simulink model "E010A5_R2_E1_energy_ton_ramp_40A_1A_20260701_003547"  (R2024b)
settings: Solver=VariableStepAuto  StartTime=0.0  StopTime=0.54e-3  MaxStep=5e-9  RelTol=1e-3
undefined symbols (not defined in the file): A_init, A_lower, A_upper, Cout, DCR_L1, DCR_L2, DCR_L3, DCR_L4, E010_AreaBleed_Enable, E010_AreaHold_Enable, E010_AreaHold_Time, E010_PulseInhibit_Count, E010_PulseInhibit_Enable, E010_PulseInhibit_Time, E010_Reentry_Band_Down, E010_ReentryGuard_Enable, E010_TonTrunc_Enable, E010_Vref, E010A5_DeltaI_Drop_Threshold_High, E010A5_IL_Sense_Gain1, E010A5_IL_Sense_Gain2, E010A5_IL_Sense_Gain3, E010A5_IL_Sense_Gain4, E010A5_R2_BudgetWindow, E010A5_R2_EnergyShaper_Enable, E010A5_R2_FirstTonLimit, E010A5_R2_PreloadTarget, E010A5_R2_ReleaseInitial, E010A5_R2_ReleaseRate, E010A5_R2_ReleaseWindow, E010A5_R2_RestoreRate, E010A5_R2_SchedulerReleaseEnable, E010A5_R2_SecondTonLimit, E010A5_R2_SoftPreloadEnable, E010A5_R2_TonBudget, E010A5_R2_TonRampMax, E010A5_R2_TonRampStep, E010A5_R2_TonRampWindow, E010A5_R2_UndershootBudget, E010A5_R2_UpperReentryBand, E010A5_R2_VoltageWindowEnable, ESR_C, IdealIQCOT_Enable, IL_adc_counts_per_A, IL_pk_limit_adc_neg, IL_pk_limit_adc_pos, Iload_final, Iload_initial, Iph, Iqcot_enable, kappa_cmd, Kiqcot, Kvc_iqcot, L, Lambda0_iqcot, Lambda_m2, rho_cmd, Ri_iqcot, t_load_step, Tblank ... (+18)
libraries: simulink x29, spsCurrentMeasurementLib x8, spsMosfetLib x8, spsSeriesRLCBranchLib x5, spsVoltageMeasurementLib x5, spsDCVoltageSourceLib x4, spsControlledCurrentSourceLib x1, spsGroundLib x1, spspowerguiLib x1
(part 1 of 2)
settings Model: Creator=zengruize  LastModifiedBy=zengruize

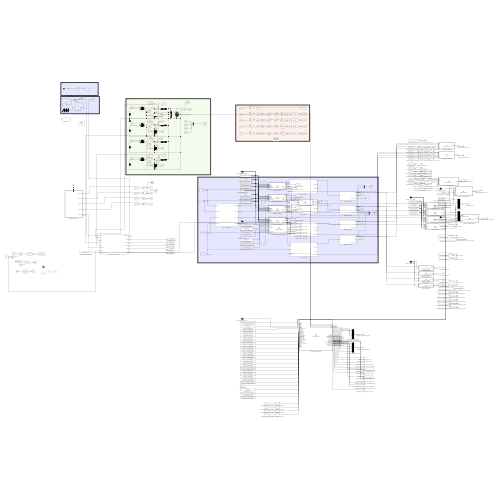
[thumbnail: Simulink's stored preview of the top-level diagram]
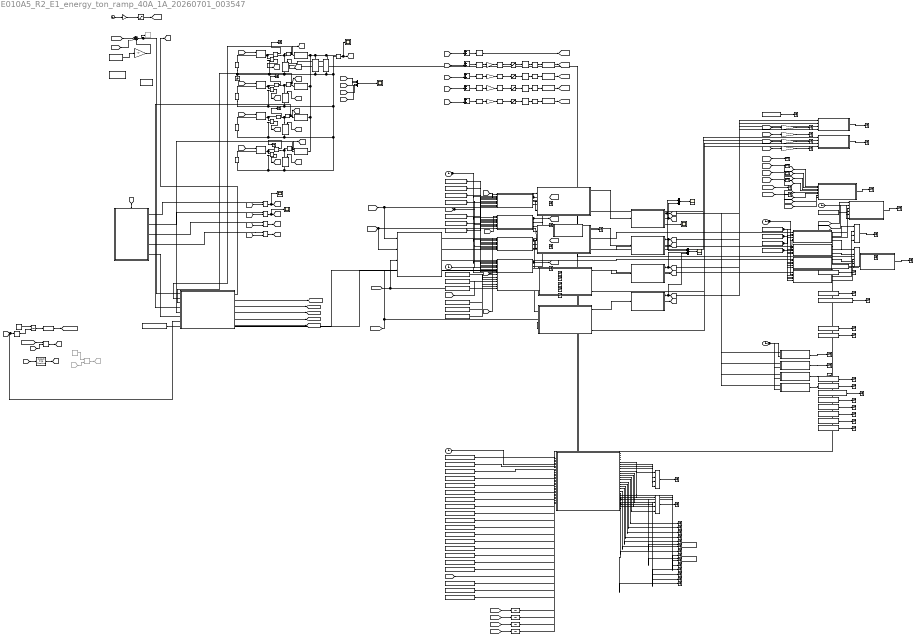
== system E010A5_R2_E1_energy_ton_ramp_40A_1A_20260701_003547 ==
  note: cot
  note: 输出电压误差比较器
  note: 功率级
  note: 软启动
  note: 采样
  Add{,1..4} (5 alike) : Sum
  Bus Creator : BusCreator  Inputs=4
  Bus Creator1 : BusCreator  Inputs=2
  Bus Creator2 : BusCreator  Inputs=4
  COT_Cell_1Phase1 : Subsystem
  COT_Cell_1Phase2 : Subsystem
  COT_Cell_1Phase3 : Subsystem
  COT_Cell_1Phase4 : Subsystem
  Clock : Clock
  Compare To Constant : simulink/Logic and Bit Operations/Compare To Constant  relop=>=  const=Tblank  OutDataTypeStr=boolean
  Constant : Constant
  Current Measurement{,1..3} (4 alike) : spsCurrentMeasurementLib/Current Measurement  PhasorSimulation=off  OutputType=Complex  PSBequivalent=0
  DC Voltage Source{,1..3} (4 alike) : spsDCVoltageSourceLib/DC Voltage Source  Amplitude=Vin  Measurements=None
  Data Type Conversion{,2..4} (4 alike) : DataTypeConversion  OutDataTypeStr=fixdt(1,14,0)  SaturateOnIntegerOverflow=off  RndMeth=Floor
  Detect Rise Positive : simulink/Logic and Bit Operations/Detect Rise Positive  vinit=0  OutDataTypeStr=boolean
  E010A5_ActiveHSPhase : MATLAB Function  TreatAsAtomicUnit=on
  E010A5_ActiveHSPhase_Term : Terminator
  E010A5_AreaBleed_Enable : Constant  Value=E010_AreaBleed_Enable
  E010A5_AreaHold_Bleed_Term : Terminator
  E010A5_AreaHold_Clock : Clock
  E010A5_AreaHold_Count_Term : Terminator
  E010A5_AreaHold_Enable : Constant  Value=E010_AreaHold_Enable
  E010A5_AreaHold_EnableProjection : MATLAB Function  TreatAsAtomicUnit=on  SystemSampleTime=Ts_ctrl
  E010A5_AreaHold_LoadStepTime : Constant  Value=t_load_step
  E010A5_AreaHold_ReentryBand : Constant  Value=E010_Reentry_Band_Down
  E010A5_AreaHold_Reset_Term : Terminator
  E010A5_AreaHold_State_Term : Terminator
  E010A5_AreaHold_Time : Constant  Value=E010_AreaHold_Time
  E010A5_AreaHold_Vref : Constant  Value=E010_Vref
  E010A5_CurrentLimitHit : MATLAB Function  TreatAsAtomicUnit=on
  E010A5_CurrentLimitHit_Term : Terminator
  E010A5_IL_Sense_Gain_Block1 : Gain  Gain=E010A5_IL_Sense_Gain1
  E010A5_IL_Sense_Gain_Block2 : Gain  Gain=E010A5_IL_Sense_Gain2
  E010A5_IL_Sense_Gain_Block3 : Gain  Gain=E010A5_IL_Sense_Gain3
  E010A5_IL_Sense_Gain_Block4 : Gain  Gain=E010A5_IL_Sense_Gain4
  E010A5_IL_Sense_Term{1..4} (4 alike) : Terminator
  E010A5_LoadCurrentStep : Step  Time=t_load_step  Before=Iload_initial  After=Iload_final  SampleTime=0
  E010A5_Load_Current_Source : spsControlledCurrentSourceLib/Controlled Current Source  Initialize=on  Source_Type=DC  Amplitude=0  Phase=0  Frequency=0  Measurements=None
  E010A5_Log_Lambda_i_Term : Terminator
  E010A5_Log_REQ1_Term : Terminator
  E010A5_Log_REQ2_Term : Terminator
  E010A5_Log_REQ3_Term : Terminator
  E010A5_Log_REQ4_Term : Terminator
  E010A5_Log_area_int_i_Term : Terminator
  E010A5_PhaseOrderError : MATLAB Function  TreatAsAtomicUnit=on  SystemSampleTime=Ts_ctrl
  E010A5_PhaseOrderError_Term : Terminator
  E010A5_PhaseOrder_Clock : Clock
  E010A5_PhaseOrder_LoadStepTime : Constant  Value=t_load_step
  E010A5_PulseInhibit1 : MATLAB Function  TreatAsAtomicUnit=on
  E010A5_PulseInhibit1_Count_Term : Terminator
  E010A5_PulseInhibit2 : MATLAB Function  TreatAsAtomicUnit=on
  E010A5_PulseInhibit2_Count_Term : Terminator
  E010A5_PulseInhibit3 : MATLAB Function  TreatAsAtomicUnit=on
  E010A5_PulseInhibit3_Count_Term : Terminator
  E010A5_PulseInhibit4 : MATLAB Function  TreatAsAtomicUnit=on
  E010A5_PulseInhibit4_Count_Term : Terminator
  E010A5_PulseInhibitState : MATLAB Function  TreatAsAtomicUnit=on
  E010A5_PulseInhibitState_Term : Terminator
  E010A5_PulseInhibit_Clock : Clock
  E010A5_PulseInhibit_Count : Constant  Value=E010_PulseInhibit_Count
  E010A5_PulseInhibit_Enable : Constant  Value=E010_PulseInhibit_Enable
  E010A5_PulseInhibit_LoadStepTime : Constant  Value=t_load_step
  E010A5_PulseInhibit_ReentryBand : Constant  Value=E010_Reentry_Band_Down
  E010A5_PulseInhibit_ReentryGuard : Constant  Value=E010_ReentryGuard_Enable
  E010A5_PulseInhibit_Time : Constant  Value=E010_PulseInhibit_Time
  E010A5_PulseInhibit_Vref : Constant  Value=E010_Vref
  E010A5_R2_BudgetWindow : Constant  Value=E010A5_R2_BudgetWindow
  E010A5_R2_EnergyShaper : MATLAB Function  TreatAsAtomicUnit=on  SystemSampleTime=Tss
  E010A5_R2_Energy_Clock : Clock
  E010A5_R2_Energy_Enable : Constant  Value=E010A5_R2_EnergyShaper_Enable
  E010A5_R2_FirstTonLimit : Constant  Value=E010A5_R2_FirstTonLimit
  E010A5_R2_LoadStepTime : Constant  Value=t_load_step
  E010A5_R2_PreloadTarget : Constant  Value=E010A5_R2_PreloadTarget
  E010A5_R2_REQAccept_Delay{1..4} (4 alike) : UnitDelay  SampleTime=Tss  HasFrameUpgradeWarning=on
  E010A5_R2_ReleaseInitial : Constant  Value=E010A5_R2_ReleaseInitial
  E010A5_R2_ReleaseRate : Constant  Value=E010A5_R2_ReleaseRate
  E010A5_R2_ReleaseWindow : Constant  Value=E010A5_R2_ReleaseWindow
  E010A5_R2_RestoreRate : Constant  Value=E010A5_R2_RestoreRate
  E010A5_R2_SchedulerReleaseEnable : Constant  Value=E010A5_R2_SchedulerReleaseEnable
  E010A5_R2_SecondTonLimit : Constant  Value=E010A5_R2_SecondTonLimit
  E010A5_R2_SoftPreloadEnable : Constant  Value=E010A5_R2_SoftPreloadEnable
  E010A5_R2_TonBudget : Constant  Value=E010A5_R2_TonBudget
  E010A5_R2_TonRampLimit_Mux : Mux
  E010A5_R2_TonRampLimit_Term : Terminator
  E010A5_R2_TonRampMax : Constant  Value=E010A5_R2_TonRampMax
  E010A5_R2_TonRampStep : Constant  Value=E010A5_R2_TonRampStep
  E010A5_R2_TonRampUsage_Mux : Mux
  E010A5_R2_TonRampUsage_Term : Terminator
  E010A5_R2_TonRampWindow : Constant  Value=E010A5_R2_TonRampWindow
  E010A5_R2_Ton_ramp_state_Term : Terminator
  E010A5_R2_UndershootBudget : Constant  Value=E010A5_R2_UndershootBudget
  E010A5_R2_UpperBand : Constant  Value=E010A5_R2_UpperReentryBand
  E010A5_R2_VoltageWindowEnable : Constant  Value=E010A5_R2_VoltageWindowEnable
  E010A5_R2_Vref : Constant  Value=E010_Vref
  E010A5_R2_area_int_restore_state_Term : Terminator
  E010A5_R2_area_int_soft_preload_count_Term : Terminator
  E010A5_R2_area_int_soft_preload_state_Term : Terminator
  E010A5_R2_controlled_reentry_active_Term : Terminator
  E010A5_R2_energy_budget_state_Term : Terminator
  E010A5_R2_reentry_energy_budget_remaining_Term : Terminator
  E010A5_R2_reentry_energy_budget_used_Term : Terminator
  E010A5_R2_reentry_energy_budget_violation_Term : Terminator
  E010A5_R2_scheduler_release_fraction_Term : Terminator
  E010A5_R2_scheduler_release_guard_violation_Term : Terminator
  E010A5_R2_scheduler_release_state_Term : Terminator
  E010A5_R2_voltage_window_release_state_Term : Terminator
  E010A5_R2_voltage_window_release_violation_Term : Terminator
  E010A5_REQRejectReason : MATLAB Function  TreatAsAtomicUnit=on
  E010A5_REQRejectReason_Term : Terminator
  E010A5_Reentry_State_Term : Terminator
  E010A5_SevereDropDetector : MATLAB Function  TreatAsAtomicUnit=on  SystemSampleTime=Ts_ctrl
  E010A5_SevereDropDetector_Clock : Clock
  E010A5_SevereDropDetector_Term : Terminator
  E010A5_SevereDropThreshold : Constant  Value=E010A5_DeltaI_Drop_Threshold_High
  E010A5_TonActual1 : MATLAB Function  TreatAsAtomicUnit=on  SystemSampleTime=Ts_ctrl
  E010A5_TonActual1_Term : Terminator
  E010A5_TonActual2 : MATLAB Function  TreatAsAtomicUnit=on  SystemSampleTime=Ts_ctrl
  E010A5_TonActual2_Term : Terminator
  E010A5_TonActual3 : MATLAB Function  TreatAsAtomicUnit=on  SystemSampleTime=Ts_ctrl
  E010A5_TonActual3_Term : Terminator
  E010A5_TonActual4 : MATLAB Function  TreatAsAtomicUnit=on  SystemSampleTime=Ts_ctrl
  E010A5_TonActual4_Term : Terminator
  E010A5_TonActual_Clock : Clock
  E010A5_TonSaved_Mux : Mux
  E010A5_TonSaved_Term : Terminator
  E010A5_TonTrunc1 : MATLAB Function  TreatAsAtomicUnit=on
  E010A5_TonTrunc2 : MATLAB Function  TreatAsAtomicUnit=on
  E010A5_TonTrunc3 : MATLAB Function  TreatAsAtomicUnit=on
  E010A5_TonTrunc4 : MATLAB Function  TreatAsAtomicUnit=on
  E010A5_TonTrunc_Clock : Clock
  E010A5_TonTrunc_Enable : Constant  Value=E010_TonTrunc_Enable
  E010A5_TonTrunc_LoadStepTime : Constant  Value=t_load_step
  E010A5_TonTrunc_Min : Constant  Value=Tton_trunc_min
  E010A5_TonTrunc_Mux : Mux
  E010A5_TonTrunc_Term : Terminator
  E010A5_TonTrunc_Window : Constant  Value=Tton_trunc_window
  E010A5_Ton_nom : Constant  Value=Ton_nom
  E010A5_Ton_nom_Term : Terminator
  E010A5_a_O_state : Constant  Value=71
  E010A5_a_O_state_Term : Terminator
  E010A5_active_phase_set : Constant  Value=[1 1 1 1]
  E010A5_active_phase_set_Term : Terminator
  E010A5_area_int_reentry_clamp : Constant  Value=0
  E010A5_area_int_reentry_clamp_Term : Terminator
  E010A5_burst_limiter_clamp_count : Constant  Value=0
  E010A5_burst_limiter_clamp_count_Term : Terminator
  E010A5_burst_limiter_fallback_reason : Constant  Value=0
  E010A5_burst_limiter_fallback_reason_Term : Terminator
  E010A5_burst_limiter_release_count : Constant  Value=0
  E010A5_burst_limiter_release_count_Term : Terminator
  E010A5_burst_limiter_state : Constant  Value=0
  E010A5_burst_limiter_state_Term : Terminator
  E010A5_burst_pulse_count_after_reentry : Constant  Value=0
  E010A5_burst_pulse_count_after_reentry_Term : Terminator
  E010A5_fallback_count : Constant  Value=0
  E010A5_fallback_count_Term : Terminator
  E010A5_fallback_reason : Constant  Value=0
  E010A5_fallback_reason_Term : Terminator
  E010A5_fallback_state : Constant  Value=0
  E010A5_fallback_state_Term : Terminator
  E010A5_recovery_Ton_ramp_usage : Constant  Value=0
  E010A5_recovery_Ton_ramp_usage_Term : Terminator
  E010A5_scheduler_release_gate_active : Constant  Value=0
  E010A5_scheduler_release_gate_active_Term : Terminator
  From31 : From  Commented=on  GotoTag=REQ
  Gain : Gain  Gain=Vo_ref / Tss
  Gain11 : Gain  Gain=205
  Gain12 : Gain  Gain=-205
  Gain13 : Gain  Gain=205
  Gain9 : Gain  Gain=-205
  GateDriver_1Phase1 : Subsystem
  GateDriver_1Phase2 : Subsystem
  GateDriver_1Phase3 : Subsystem
  GateDriver_1Phase4 : Subsystem
  Goto26 : Goto  Commented=on  GotoTag=tr
  Ground : spsGroundLib/Ground  LConnTagsString=a
  IHS_Terminator{1..4} (4 alike) : Terminator
  IL_Measurement{1..4} (4 alike) : spsCurrentMeasurementLib/Current Measurement  PhasorSimulation=off  OutputType=Complex  PSBequivalent=0
  IQCOT_Ton_Adapter : Subsystem
  IdealIQCOT_Enable_Constant : Constant  Value=IdealIQCOT_Enable
  Ideal_Digital_IQCOT_Request : Subsystem
  Integrator : Integrator  ExternalReset=rising
  Logical Operator{,1..4} (5 alike) : Logic  AllPortsSameDT=off  OutDataTypeStr=boolean
  Logical Operator5 : Logic  Commented=on  AllPortsSameDT=off  OutDataTypeStr=boolean
  Memory : Memory
  Mosfet{,1..3} (4 alike) : spsMosfetLib/Mosfet  Ron=Ron_HS  Lon=0  Rd=Rd_body  Vfd=Vfd_body  IC=0  Rs=Rs_snubber  Cs=Cs_snubber  Measurements=on
  Mosfet{4..7} (4 alike) : spsMosfetLib/Mosfet  Ron=Ron_LS  Lon=0  Rd=Rd_body  Vfd=Vfd_body  IC=0  Rs=Rs_snubber  Cs=Cs_snubber  Measurements=on
  OnDelay : Subsystem
  PhaseScheduler_4Phase : Subsystem  TreatAsAtomicUnit=on
  Pulse Generator : DiscretePulseGenerator  Commented=on  PulseType=Time based  Period=Tblank  PulseWidth=5
  Quantizer{1..4} (4 alike) : Quantizer  QuantizationInterval=1
  Relay : Relay  Commented=through  OnSwitchValue=Vhys/2  OffSwitchValue=-Vhys/2
  Saturation{,1,3..4} (4 alike) : Saturate  UpperLimit=8191  LowerLimit=-8191
  Saturation2 : Saturate  UpperLimit=Vo_ref  LowerLimit=0
  Scope{,1..6} (7 alike) : Scope
  Series RLC Branch : spsSeriesRLCBranchLib/Series RLC Branch  LConnTagsString=__new0  RConnTagsString=__new0  BranchType=RL  Resistance=DCR_L1  Inductance=L  SetiL0=off  InitialCurrent=0  Capacitance=1e-6  Setx0=off  InitialVoltage=0  Measurements=None
  Series RLC Branch1 : spsSeriesRLCBranchLib/Series RLC Branch  LConnTagsString=__new0  RConnTagsString=__new0  BranchType=RL  Resistance=DCR_L2  Inductance=L  SetiL0=off  InitialCurrent=0  Capacitance=1e-6  Setx0=off  InitialVoltage=0  Measurements=None
  Series RLC Branch2 : spsSeriesRLCBranchLib/Series RLC Branch  LConnTagsString=__new0  RConnTagsString=__new0  BranchType=RL  Resistance=DCR_L3  Inductance=L  SetiL0=off  InitialCurrent=0  Capacitance=1e-6  Setx0=off  InitialVoltage=0  Measurements=None
  Series RLC Branch3 : spsSeriesRLCBranchLib/Series RLC Branch  LConnTagsString=__new0  RConnTagsString=__new0  BranchType=RL  Resistance=DCR_L4  Inductance=L  SetiL0=off  InitialCurrent=0  Capacitance=1e-6  Setx0=off  InitialVoltage=0  Measurements=None
  Series RLC Branch4 : spsSeriesRLCBranchLib/Series RLC Branch  LConnTagsString=__new0  RConnTagsString=__new0  BranchType=RC  Resistance=ESR_C  Inductance=1e-3  SetiL0=off  InitialCurrent=0  Capacitance=Cout  Setx0=on  InitialVoltage=Vo_ref  Measurements=None
  Sum : Sum  Inputs=|+--
  Transport Delay{1..4} (4 alike) : TransportDelay  DelayTime=5/25000000
  VCOT_Ramp_Gain : Gain  Gain=Vcot_ramp_enable * Vcot_ramp_amp
  VCOT_Ramp_Unit : simulink/Sources/Repeating Sequence  rep_seq_t=[0 Tslot]  rep_seq_y=[0 1]
  Voltage Measurement{,1..4} (5 alike) : spsVoltageMeasurementLib/Voltage Measurement  PhasorSimulation=off  OutputType=Complex  PSBequivalent=0
  Zero-Order Hold{1..4,19..23} (9 alike) : ZeroOrderHold  SampleTime=1/25000000
  powergui : spspowerguiLib/powergui  Priority=1  SimulationMode=Discrete  SampleTime=2e-9  frequency=60  Iterations=50  frequencyindice=0  Pbase=100e6  ErrMax=1e-4  UnitsV=kV  UnitsW=MW  buscounter=0  FunctionMessages=off  echomessages=off  EnableUseOfTLC=off  CurrentSourceSwitches=off  DisableSnubberDevices=off  DisableRonSwitches=off  DisableVfSwitches=off  DisplayEquations=off  AutomaticDiscreteSolvers=off  SolverType=Tustin/Backward Euler (TBE)  Interpol=off  ExternalGateDelay=off  methode=off  Ts=100  x0status=blocks  SPID=on  SwTol=0  HookPort=off  NonlinearTolerance=1e-4  nMaxIteration=100  ContinueOnMaxIteration=off  RestoreLinks=warning  ResistiveCurrentMeasurement=off  Frange=[0:2:500]  Ylog=off  Xlog=on  ShowGrid=off  save=off  variable=ZData  structure=0  ZoomFFT=off  StartTime=0.0  cycles=1  DisplayStyle=1  fundamental=60  FreqAxis=off  MaxFrequency=1000  frequencyindicesteady=1  RmsSteady=1  display=off
  wires:
  [QH1] -> Mosfet/1
  [QH4] -> Mosfet3/1
  [QH2] -> Mosfet1/1
  [QH3] -> Mosfet2/1
  [QL1] -> Mosfet4/1
  [QL2] -> Mosfet5/1
  [QL3] -> Mosfet6/1
  [QL4] -> Mosfet7/1
  Voltage Measurement2/1 -> [SW2]  "SW2"
  Voltage Measurement3/1 -> [SW3]  "SW3"
  Voltage Measurement1/1 -> [SW1]  "SW1"
  Voltage Measurement4/1 -> [SW4]  "SW4"
  GateDriver_1Phase1/1(QHi) -> Bus Creator1/1, [QH1], Bus Creator2/1, E010A5_ActiveHSPhase/1(qh1), E010A5_TonActual1/1(qh)  "QH1"
  GateDriver_1Phase2/1(QHi) -> Bus Creator2/2, [QH2], E010A5_ActiveHSPhase/2(qh2), E010A5_TonActual2/1(qh)  "QH2"
  GateDriver_1Phase3/1(QHi) -> Bus Creator2/3, [QH3], E010A5_ActiveHSPhase/3(qh3), E010A5_TonActual3/1(qh)  "QH3"
  GateDriver_1Phase4/1(QHi) -> Bus Creator2/4, [QH4], E010A5_ActiveHSPhase/4(qh4), E010A5_TonActual4/1(qh)  "QH4"
  GateDriver_1Phase1/2(QLi) -> Bus Creator1/2, [QL1]  "QL1"
  GateDriver_1Phase2/2(QLi) -> [QL2]  "QL2"
  GateDriver_1Phase3/2(QLi) -> [QL3]  "QL3"
  GateDriver_1Phase4/2(QLi) -> [QL4]  "QL4"
  COT_Cell_1Phase1/1(Qi) -> GateDriver_1Phase1/1(Qi)
  COT_Cell_1Phase2/1(Qi) -> GateDriver_1Phase2/1(Qi)
  COT_Cell_1Phase3/1(Qi) -> GateDriver_1Phase3/1(Qi)
  COT_Cell_1Phase4/1(Qi) -> GateDriver_1Phase4/1(Qi)
  GateDriver_1Phase1/3(ShootThrough_i) -> Scope1/1
  Bus Creator/1 -> Scope2/1
  [SW1] -> Bus Creator/1
  [SW2] -> Bus Creator/2
  [SW3] -> Bus Creator/3
  [SW4] -> Bus Creator/4
  Bus Creator1/1 -> Scope3/1
  Saturation2/1 -> [Vref_soft]
  Gain/1 -> Saturation2/1
  Clock/1 -> Gain/1
  Voltage Measurement/1 -> Scope/1, [Vout]  "Vout"
  [Vref_soft] -> Sum/1
  [Vo_sample] -> Sum/2
  Sum/1 -> Ideal_Digital_IQCOT_Request/1(e_v), Relay/1  "e_v"
  Constant/1 -> Integrator/1
  Integrator/1 -> Compare To Constant/1
  Compare To Constant/1 -> [GlobalReady]  "Allow"
  [GlobalReady] -> Logical Operator/1
  [REQ] -> Logical Operator/2
  Logical Operator/1 -> [Allow]
  [Allow] -> Detect Rise Positive/1
  Detect Rise Positive/1 -> [tr]
  [tr] -> PhaseScheduler_4Phase/Trigger  "tr"
  PhaseScheduler_4Phase/1(phase_en1) -> Logical Operator1/1
  [tr] -> Logical Operator1/2
  PhaseScheduler_4Phase/2(phase_en2) -> Logical Operator2/1
  [tr] -> Logical Operator2/2
  PhaseScheduler_4Phase/3(phase_en3) -> Logical Operator3/1
  [tr] -> Logical Operator3/2
  PhaseScheduler_4Phase/4(phase_en4) -> Logical Operator4/1
  [tr] -> Logical Operator4/2
  Logical Operator1/1 -> Scope4/1, [tr1]  "tr1"
  Logical Operator2/1 -> Scope5/1, [tr2]  "tr2"
  Logical Operator3/1 -> [tr3]  "tr3"
  Logical Operator4/1 -> [tr4]  "tr4"
  [IL_sample1] -> COT_Cell_1Phase1/2(ILi), IQCOT_Ton_Adapter/1(IL_sample1)  "IL_sample1"
  [IL_sample2] -> IQCOT_Ton_Adapter/2(IL_sample2), COT_Cell_1Phase2/2(ILi)  "IL_sample2"
  [IL_sample3] -> IQCOT_Ton_Adapter/3(IL_sample3), COT_Cell_1Phase3/2(ILi)  "IL_sample3"
  [IL_sample4] -> IQCOT_Ton_Adapter/4(IL_sample4), COT_Cell_1Phase4/2(ILi)  "IL_sample4"
  [tr] -> Memory/1, Ideal_Digital_IQCOT_Request/7(tr_reset)  "tr_reset"
  Memory/1 -> Integrator/2
  Logical Operator5/1 -> Goto26/1
  Pulse Generator/1 -> Logical Operator5/1
  From31/1 -> Logical Operator5/2
  Bus Creator2/1 -> Scope6/1
  IL_Measurement1/1 -> [IL1], Ideal_Digital_IQCOT_Request/2(IL1)  "IL1"
  IL_Measurement2/1 -> [IL2], Ideal_Digital_IQCOT_Request/3(IL2)  "IL2"
  IL_Measurement3/1 -> [IL3], Ideal_Digital_IQCOT_Request/4(IL3)  "IL3"
  IL_Measurement4/1 -> [IL4], Ideal_Digital_IQCOT_Request/5(IL4)  "IL4"
  Current Measurement/1 -> IHS_Terminator1/1
  Current Measurement1/1 -> IHS_Terminator2/1
  Current Measurement2/1 -> IHS_Terminator3/1
  Current Measurement3/1 -> IHS_Terminator4/1
  Zero-Order Hold23/1 -> Gain13/1
  Zero-Order Hold20/1 -> Gain9/1
  Zero-Order Hold3/1 -> Data Type Conversion3/1
  Zero-Order Hold4/1 -> Data Type Conversion2/1
  Saturation4/1 -> Transport Delay4/1
  Zero-Order Hold1/1 -> Data Type Conversion/1
  [IL3] -> Add3/2
  Add3/1 -> Zero-Order Hold22/1
  Quantizer1/1 -> Saturation/1
  Quantizer4/1 -> Saturation4/1
  Gain12/1 -> Quantizer3/1
  [IL4] -> Add4/2
  Add/1 -> Zero-Order Hold19/1
  Data Type Conversion/1 -> [IL_sample1]
  Data Type Conversion2/1 -> [IL_sample4]
  Add4/1 -> Zero-Order Hold23/1
  Transport Delay3/1 -> Zero-Order Hold3/1
  Saturation3/1 -> Transport Delay3/1
  Add1/1 -> Zero-Order Hold20/1
  [IL1] -> Add1/2
  Transport Delay4/1 -> Zero-Order Hold4/1
  Zero-Order Hold21/1 -> Gain11/1
  Data Type Conversion3/1 -> [IL_sample3]
  Gain9/1 -> Quantizer1/1
  Gain11/1 -> Quantizer2/1
  Saturation/1 -> Transport Delay1/1
  [IL2] -> Add2/2
  Transport Delay2/1 -> Zero-Order Hold2/1
  Zero-Order Hold19/1 -> [Vo_sample]
  Gain13/1 -> Quantizer4/1
  Quantizer3/1 -> Saturation3/1
  Data Type Conversion4/1 -> [IL_sample2]
  Zero-Order Hold2/1 -> Data Type Conversion4/1
  Add2/1 -> Zero-Order Hold21/1
  Transport Delay1/1 -> Zero-Order Hold1/1
  [Vout] -> Add/2
  Saturation1/1 -> Transport Delay2/1
  Zero-Order Hold22/1 -> Gain12/1
  Quantizer2/1 -> Saturation1/1
  VCOT_Ramp_Unit/1 -> VCOT_Ramp_Gain/1
  VCOT_Ramp_Gain/1 -> Sum/3  "Vcot_ramp"
  PhaseScheduler_4Phase/5(phase_idx) -> Ideal_Digital_IQCOT_Request/6(phase_idx)  "phase_idx"
  Ideal_Digital_IQCOT_Request/1(REQ_iqcot) -> [REQ]  "REQ_iqcot"
  Ideal_Digital_IQCOT_Request/2(A_iqcot) -> [A_iqcot]  "A_iqcot"
  Ideal_Digital_IQCOT_Request/3(Lambda_i) -> [Lambda_i]  "Lambda_i"
  Ideal_Digital_IQCOT_Request/4(h_iqcot) -> [h_iqcot]  "h_iqcot"
  Ideal_Digital_IQCOT_Request/5(IL_sel) -> [IL_sel]  "IL_sel"
  Ideal_Digital_IQCOT_Request/6(vc_ctrl) -> [vc_ctrl]  "vc_ctrl"
  E010A5_LoadCurrentStep/1 -> E010A5_Load_Current_Source/1, E010A5_SevereDropDetector/1(iload)  "Iload"
  E010A5_active_phase_set/1 -> E010A5_active_phase_set_Term/1  "active_phase_set"
  [IL1] -> E010A5_IL_Sense_Gain_Block1/1
  E010A5_IL_Sense_Gain_Block1/1 -> E010A5_IL_Sense_Term1/1  "IL_sense1"
  [IL2] -> E010A5_IL_Sense_Gain_Block2/1
  E010A5_IL_Sense_Gain_Block2/1 -> E010A5_IL_Sense_Term2/1  "IL_sense2"
  [IL3] -> E010A5_IL_Sense_Gain_Block3/1
  E010A5_IL_Sense_Gain_Block3/1 -> E010A5_IL_Sense_Term3/1  "IL_sense3"
  [IL4] -> E010A5_IL_Sense_Gain_Block4/1
  E010A5_IL_Sense_Gain_Block4/1 -> E010A5_IL_Sense_Term4/1  "IL_sense4"
  [tr1] -> E010A5_Log_REQ1_Term/1  "REQ1"
  [tr2] -> E010A5_Log_REQ2_Term/1  "REQ2"
  [tr3] -> E010A5_Log_REQ3_Term/1  "REQ3"
  [tr4] -> E010A5_Log_REQ4_Term/1  "REQ4"
  [Lambda_i] -> E010A5_Log_Lambda_i_Term/1  "Lambda_i"
  [A_iqcot] -> E010A5_Log_area_int_i_Term/1  "area_int_i"
  E010A5_ActiveHSPhase/1(active_phase) -> E010A5_ActiveHSPhase_Term/1  "active_HS_phase"
  COT_Cell_1Phase1/4(CurrentLimit_i) -> E010A5_CurrentLimitHit/1(u1)
  COT_Cell_1Phase2/4(CurrentLimit_i) -> E010A5_CurrentLimitHit/2(u2)
  COT_Cell_1Phase3/4(CurrentLimit_i) -> E010A5_CurrentLimitHit/3(u3)
  COT_Cell_1Phase4/4(CurrentLimit_i) -> E010A5_CurrentLimitHit/4(u4)
  E010A5_CurrentLimitHit/1(y) -> E010A5_CurrentLimitHit_Term/1  "current_limit_hit"
  IQCOT_Ton_Adapter/1(Ton_iqcot1) -> E010A5_TonTrunc1/1(ton_in)  "Ton_iqcot1"
  E010A5_TonTrunc_Clock/1 -> E010A5_TonTrunc1/2(t), E010A5_TonTrunc2/2(t), E010A5_TonTrunc3/2(t), E010A5_TonTrunc4/2(t)
  E010A5_TonTrunc_LoadStepTime/1 -> E010A5_TonTrunc1/3(t_step), E010A5_TonTrunc2/3(t_step), E010A5_TonTrunc3/3(t_step), E010A5_TonTrunc4/3(t_step)
  E010A5_TonTrunc_Window/1 -> E010A5_TonTrunc1/4(t_window), E010A5_TonTrunc2/4(t_window), E010A5_TonTrunc3/4(t_window), E010A5_TonTrunc4/4(t_window)
  E010A5_TonTrunc_Min/1 -> E010A5_TonTrunc1/5(t_min), E010A5_TonTrunc2/5(t_min), E010A5_TonTrunc3/5(t_min), E010A5_TonTrunc4/5(t_min)
  E010A5_TonTrunc_Enable/1 -> E010A5_TonTrunc1/6(enable), E010A5_TonTrunc2/6(enable), E010A5_TonTrunc3/6(enable), E010A5_TonTrunc4/6(enable)
  E010A5_TonTrunc1/1(ton_out) -> E010A5_R2_EnergyShaper/1(ton1)  "Ton_cmd1"
  E010A5_TonTrunc1/2(trunc_active) -> E010A5_TonTrunc_Mux/1
  E010A5_TonTrunc1/3(ton_saved) -> E010A5_TonSaved_Mux/1
  IQCOT_Ton_Adapter/2(Ton_iqcot2) -> E010A5_TonTrunc2/1(ton_in)  "Ton_iqcot2"
  E010A5_TonTrunc2/1(ton_out) -> E010A5_R2_EnergyShaper/2(ton2)  "Ton_cmd2"
  E010A5_TonTrunc2/2(trunc_active) -> E010A5_TonTrunc_Mux/2
  E010A5_TonTrunc2/3(ton_saved) -> E010A5_TonSaved_Mux/2
  IQCOT_Ton_Adapter/3(Ton_iqcot3) -> E010A5_TonTrunc3/1(ton_in)  "Ton_iqcot3"
  E010A5_TonTrunc3/1(ton_out) -> E010A5_R2_EnergyShaper/3(ton3)  "Ton_cmd3"
  E010A5_TonTrunc3/2(trunc_active) -> E010A5_TonTrunc_Mux/3
  E010A5_TonTrunc3/3(ton_saved) -> E010A5_TonSaved_Mux/3
  IQCOT_Ton_Adapter/4(Ton_iqcot4) -> E010A5_TonTrunc4/1(ton_in)  "Ton_iqcot4"
  E010A5_TonTrunc4/1(ton_out) -> E010A5_R2_EnergyShaper/4(ton4)  "Ton_cmd4"
  E010A5_TonTrunc4/2(trunc_active) -> E010A5_TonTrunc_Mux/4
  E010A5_TonTrunc4/3(ton_saved) -> E010A5_TonSaved_Mux/4
  E010A5_TonTrunc_Mux/1 -> E010A5_TonTrunc_Term/1  "Ton_trunc_i"
  E010A5_TonSaved_Mux/1 -> E010A5_TonSaved_Term/1  "Ton_saved_i"
  [tr1] -> E010A5_PulseInhibit1/1(tr_in)
  E010A5_PulseInhibit_Clock/1 -> E010A5_PulseInhibit1/2(t), E010A5_PulseInhibit2/2(t), E010A5_PulseInhibit3/2(t), E010A5_PulseInhibit4/2(t)
  E010A5_PulseInhibit_LoadStepTime/1 -> E010A5_PulseInhibit1/3(t_step), E010A5_PulseInhibit2/3(t_step), E010A5_PulseInhibit3/3(t_step), E010A5_PulseInhibit4/3(t_step)
  E010A5_PulseInhibit_Time/1 -> E010A5_PulseInhibit1/4(t_window), E010A5_PulseInhibit2/4(t_window), E010A5_PulseInhibit3/4(t_window), E010A5_PulseInhibit4/4(t_window)
  E010A5_PulseInhibit_Count/1 -> E010A5_PulseInhibit1/5(count_max), E010A5_PulseInhibit2/5(count_max), E010A5_PulseInhibit3/5(count_max), E010A5_PulseInhibit4/5(count_max)
  E010A5_PulseInhibit_Enable/1 -> E010A5_PulseInhibit1/6(enable), E010A5_PulseInhibit2/6(enable), E010A5_PulseInhibit3/6(enable), E010A5_PulseInhibit4/6(enable)
  [Vout] -> E010A5_PulseInhibit1/7(vout), E010A5_PulseInhibit2/7(vout), E010A5_PulseInhibit3/7(vout), E010A5_PulseInhibit4/7(vout)
  E010A5_PulseInhibit_Vref/1 -> E010A5_PulseInhibit1/8(vref), E010A5_PulseInhibit2/8(vref), E010A5_PulseInhibit3/8(vref), E010A5_PulseInhibit4/8(vref)
  E010A5_PulseInhibit_ReentryBand/1 -> E010A5_PulseInhibit1/9(reentry_band), E010A5_PulseInhibit2/9(reentry_band), E010A5_PulseInhibit3/9(reentry_band), E010A5_PulseInhibit4/9(reentry_band)
  E010A5_PulseInhibit_ReentryGuard/1 -> E010A5_PulseInhibit1/10(guard_enable), E010A5_PulseInhibit2/10(guard_enable), E010A5_PulseInhibit3/10(guard_enable), E010A5_PulseInhibit4/10(guard_enable)
  E010A5_PulseInhibit1/1(tr_out) -> COT_Cell_1Phase1/1(tri), [REQ_accept1]  "REQ_accept1"
  E010A5_PulseInhibit1/2(inhibit_active) -> E010A5_PulseInhibitState/1(u1)
  E010A5_PulseInhibit1/3(inhibit_count) -> E010A5_PulseInhibit1_Count_Term/1  "pulse_inhibit_count1"
  [tr2] -> E010A5_PulseInhibit2/1(tr_in)
  E010A5_PulseInhibit2/1(tr_out) -> COT_Cell_1Phase2/1(tri), [REQ_accept2]  "REQ_accept2"
  E010A5_PulseInhibit2/2(inhibit_active) -> E010A5_PulseInhibitState/2(u2)
  E010A5_PulseInhibit2/3(inhibit_count) -> E010A5_PulseInhibit2_Count_Term/1  "pulse_inhibit_count2"
  [tr3] -> E010A5_PulseInhibit3/1(tr_in)
  E010A5_PulseInhibit3/1(tr_out) -> COT_Cell_1Phase3/1(tri), [REQ_accept3]  "REQ_accept3"
  E010A5_PulseInhibit3/2(inhibit_active) -> E010A5_PulseInhibitState/3(u3)
  E010A5_PulseInhibit3/3(inhibit_count) -> E010A5_PulseInhibit3_Count_Term/1  "pulse_inhibit_count3"
  [tr4] -> E010A5_PulseInhibit4/1(tr_in)
  E010A5_PulseInhibit4/1(tr_out) -> COT_Cell_1Phase4/1(tri), [REQ_accept4]  "REQ_accept4"
  E010A5_PulseInhibit4/2(inhibit_active) -> E010A5_PulseInhibitState/4(u4)
  E010A5_PulseInhibit4/3(inhibit_count) -> E010A5_PulseInhibit4_Count_Term/1  "pulse_inhibit_count4"
  E010A5_PulseInhibitState/1(y) -> E010A5_PulseInhibitState_Term/1  "pulse_inhibit_state"
  IdealIQCOT_Enable_Constant/1 -> E010A5_AreaHold_EnableProjection/1(enable_in)
  E010A5_AreaHold_Clock/1 -> E010A5_AreaHold_EnableProjection/2(t)
  E010A5_AreaHold_LoadStepTime/1 -> E010A5_AreaHold_EnableProjection/3(t_step)
  E010A5_AreaHold_Time/1 -> E010A5_AreaHold_EnableProjection/4(t_hold)
  E010A5_AreaHold_Enable/1 -> E010A5_AreaHold_EnableProjection/5(hold_enable)
  [Vout] -> E010A5_AreaHold_EnableProjection/6(vout)
  E010A5_AreaHold_Vref/1 -> E010A5_AreaHold_EnableProjection/7(vref)
  E010A5_AreaHold_ReentryBand/1 -> E010A5_AreaHold_EnableProjection/8(reentry_band)
  E010A5_AreaBleed_Enable/1 -> E010A5_AreaHold_EnableProjection/9(bleed_enable)
  E010A5_AreaHold_EnableProjection/1(enable_out) -> Ideal_Digital_IQCOT_Request/8(enable)
  E010A5_AreaHold_EnableProjection/2(hold_state) -> E010A5_AreaHold_State_Term/1  "area_hold_state"
  E010A5_AreaHold_EnableProjection/3(hold_count) -> E010A5_AreaHold_Count_Term/1  "area_hold_count"
  E010A5_AreaHold_EnableProjection/4(reset_count) -> E010A5_AreaHold_Reset_Term/1  "area_reset_count"
  E010A5_AreaHold_EnableProjection/5(bleed_count) -> E010A5_AreaHold_Bleed_Term/1  "area_bleed_count"
  E010A5_AreaHold_EnableProjection/6(reentry_state) -> E010A5_Reentry_State_Term/1  "reentry_state"
  E010A5_R2_Energy_Clock/1 -> E010A5_R2_EnergyShaper/5(t)
  E010A5_R2_LoadStepTime/1 -> E010A5_R2_EnergyShaper/6(t_step)
  E010A5_R2_Energy_Enable/1 -> E010A5_R2_EnergyShaper/7(enable)
  E010A5_R2_BudgetWindow/1 -> E010A5_R2_EnergyShaper/8(budget_window)
  E010A5_R2_TonBudget/1 -> E010A5_R2_EnergyShaper/9(ton_budget)
  E010A5_R2_FirstTonLimit/1 -> E010A5_R2_EnergyShaper/10(first_lim)
  E010A5_R2_SecondTonLimit/1 -> E010A5_R2_EnergyShaper/11(second_lim)
  E010A5_R2_TonRampStep/1 -> E010A5_R2_EnergyShaper/12(ton_step)
  E010A5_R2_TonRampWindow/1 -> E010A5_R2_EnergyShaper/13(ramp_window)
  E010A5_R2_TonRampMax/1 -> E010A5_R2_EnergyShaper/14(max_ton)
  E010A5_R2_SoftPreloadEnable/1 -> E010A5_R2_EnergyShaper/15(soft_enable)
  E010A5_R2_PreloadTarget/1 -> E010A5_R2_EnergyShaper/16(preload_target)
  E010A5_R2_RestoreRate/1 -> E010A5_R2_EnergyShaper/17(restore_rate)
  E010A5_R2_SchedulerReleaseEnable/1 -> E010A5_R2_EnergyShaper/18(sched_enable)
  E010A5_R2_ReleaseInitial/1 -> E010A5_R2_EnergyShaper/19(release_initial)
  E010A5_R2_ReleaseRate/1 -> E010A5_R2_EnergyShaper/20(release_rate)
  E010A5_R2_ReleaseWindow/1 -> E010A5_R2_EnergyShaper/21(release_window)
  E010A5_R2_VoltageWindowEnable/1 -> E010A5_R2_EnergyShaper/22(voltage_enable)
  [Vout] -> E010A5_R2_EnergyShaper/23(vout)
  E010A5_R2_Vref/1 -> E010A5_R2_EnergyShaper/24(vref)
  E010A5_R2_UpperBand/1 -> E010A5_R2_EnergyShaper/25(upper_band)
  E010A5_R2_UndershootBudget/1 -> E010A5_R2_EnergyShaper/26(undershoot_budget)
  [REQ_accept1] -> E010A5_R2_REQAccept_Delay1/1
  E010A5_R2_REQAccept_Delay1/1 -> E010A5_R2_EnergyShaper/27(req1)
  [REQ_accept2] -> E010A5_R2_REQAccept_Delay2/1
  E010A5_R2_REQAccept_Delay2/1 -> E010A5_R2_EnergyShaper/28(req2)
  [REQ_accept3] -> E010A5_R2_REQAccept_Delay3/1
  E010A5_R2_REQAccept_Delay3/1 -> E010A5_R2_EnergyShaper/29(req3)
  [REQ_accept4] -> E010A5_R2_REQAccept_Delay4/1
  E010A5_R2_REQAccept_Delay4/1 -> E010A5_R2_EnergyShaper/30(req4)
  E010A5_R2_EnergyShaper/1(ton1o) -> COT_Cell_1Phase1/3(Ton_iqcot1)  "Ton_cmd1"
  E010A5_R2_EnergyShaper/5(u1) -> E010A5_R2_TonRampUsage_Mux/1
  E010A5_R2_EnergyShaper/9(l1) -> E010A5_R2_TonRampLimit_Mux/1
  E010A5_R2_EnergyShaper/2(ton2o) -> COT_Cell_1Phase2/3(Ton_iqcot2)  "Ton_cmd2"
  E010A5_R2_EnergyShaper/6(u2) -> E010A5_R2_TonRampUsage_Mux/2
  E010A5_R2_EnergyShaper/10(l2) -> E010A5_R2_TonRampLimit_Mux/2
  E010A5_R2_EnergyShaper/3(ton3o) -> COT_Cell_1Phase3/3(Ton_iqcot3)  "Ton_cmd3"
  E010A5_R2_EnergyShaper/7(u3) -> E010A5_R2_TonRampUsage_Mux/3
  E010A5_R2_EnergyShaper/11(l3) -> E010A5_R2_TonRampLimit_Mux/3
  E010A5_R2_EnergyShaper/4(ton4o) -> COT_Cell_1Phase4/3(Ton_iqcot4)  "Ton_cmd4"
  E010A5_R2_EnergyShaper/8(u4) -> E010A5_R2_TonRampUsage_Mux/4
  E010A5_R2_EnergyShaper/12(l4) -> E010A5_R2_TonRampLimit_Mux/4
  E010A5_R2_TonRampUsage_Mux/1 -> E010A5_R2_TonRampUsage_Term/1  "Ton_ramp_usage"
  E010A5_R2_TonRampLimit_Mux/1 -> E010A5_R2_TonRampLimit_Term/1  "Ton_ramp_limit_i"
  E010A5_R2_EnergyShaper/13(ton_state) -> E010A5_R2_Ton_ramp_state_Term/1  "Ton_ramp_state"
  E010A5_R2_EnergyShaper/14(budget_state) -> E010A5_R2_energy_budget_state_Term/1  "energy_budget_state"
  E010A5_R2_EnergyShaper/15(budget_used) -> E010A5_R2_reentry_energy_budget_used_Term/1  "reentry_energy_budget_used"
  E010A5_R2_EnergyShaper/16(budget_remaining) -> E010A5_R2_reentry_energy_budget_remaining_Term/1  "reentry_energy_budget_remaining"
  E010A5_R2_EnergyShaper/17(budget_violation) -> E010A5_R2_reentry_energy_budget_violation_Term/1  "reentry_energy_budget_violation"
  E010A5_R2_EnergyShaper/18(soft_state) -> E010A5_R2_area_int_soft_preload_state_Term/1  "area_int_soft_preload_state"
  E010A5_R2_EnergyShaper/19(soft_count) -> E010A5_R2_area_int_soft_preload_count_Term/1  "area_int_soft_preload_count"
  E010A5_R2_EnergyShaper/20(restore_state) -> E010A5_R2_area_int_restore_state_Term/1  "area_int_restore_state"
  E010A5_R2_EnergyShaper/21(sched_state) -> E010A5_R2_scheduler_release_state_Term/1  "scheduler_release_state"
  E010A5_R2_EnergyShaper/22(sched_fraction) -> E010A5_R2_scheduler_release_fraction_Term/1, [E010A5_R2_scheduler_release_fraction]  "scheduler_release_fraction"
  E010A5_R2_EnergyShaper/23(sched_guard_violation) -> E010A5_R2_scheduler_release_guard_violation_Term/1  "scheduler_release_guard_violation"
  E010A5_R2_EnergyShaper/24(voltage_state) -> E010A5_R2_voltage_window_release_state_Term/1, [E010A5_R2_voltage_window_state]  "voltage_window_release_state"
  E010A5_R2_EnergyShaper/25(voltage_violation) -> E010A5_R2_voltage_window_release_violation_Term/1  "voltage_window_release_violation"
  E010A5_R2_EnergyShaper/26(controlled_active) -> E010A5_R2_controlled_reentry_active_Term/1  "controlled_reentry_active"
  E010A5_Ton_nom/1 -> E010A5_Ton_nom_Term/1  "Ton_nom"
  E010A5_burst_limiter_state/1 -> E010A5_burst_limiter_state_Term/1  "burst_limiter_state"
  E010A5_area_int_reentry_clamp/1 -> E010A5_area_int_reentry_clamp_Term/1  "area_int_reentry_clamp"
  E010A5_burst_limiter_clamp_count/1 -> E010A5_burst_limiter_clamp_count_Term/1  "burst_limiter_clamp_count"
  E010A5_burst_limiter_release_count/1 -> E010A5_burst_limiter_release_count_Term/1  "burst_limiter_release_count"
  E010A5_burst_limiter_fallback_reason/1 -> E010A5_burst_limiter_fallback_reason_Term/1  "burst_limiter_fallback_reason"
  E010A5_recovery_Ton_ramp_usage/1 -> E010A5_recovery_Ton_ramp_usage_Term/1  "recovery_Ton_ramp_usage"
  E010A5_scheduler_release_gate_active/1 -> E010A5_scheduler_release_gate_active_Term/1  "scheduler_release_gate_active"
  [tr1] -> E010A5_REQRejectReason/1(r1)
  [REQ_accept1] -> E010A5_REQRejectReason/5(a1)
  [tr2] -> E010A5_REQRejectReason/2(r2)
  [REQ_accept2] -> E010A5_REQRejectReason/6(a2)
  [tr3] -> E010A5_REQRejectReason/3(r3)
  [REQ_accept3] -> E010A5_REQRejectReason/7(a3)
  [tr4] -> E010A5_REQRejectReason/4(r4)
  [REQ_accept4] -> E010A5_REQRejectReason/8(a4)
  E010A5_REQRejectReason/1(reason) -> E010A5_REQRejectReason_Term/1  "REQ_reject_reason"
  [REQ_accept1] -> E010A5_PhaseOrderError/1(a1)
  [REQ_accept2] -> E010A5_PhaseOrderError/2(a2)
  [REQ_accept3] -> E010A5_PhaseOrderError/3(a3)
  [REQ_accept4] -> E010A5_PhaseOrderError/4(a4)
  E010A5_PhaseOrder_Clock/1 -> E010A5_PhaseOrderError/5(t)
  E010A5_PhaseOrder_LoadStepTime/1 -> E010A5_PhaseOrderError/6(t_step)
  E010A5_PhaseOrderError/1(err) -> E010A5_PhaseOrderError_Term/1  "phase_order_error"
  E010A5_SevereDropDetector_Clock/1 -> E010A5_SevereDropDetector/2(t)
  E010A5_SevereDropThreshold/1 -> E010A5_SevereDropDetector/3(threshold)
  E010A5_SevereDropDetector/1(detected) -> E010A5_SevereDropDetector_Term/1  "severe_drop_detected"
  E010A5_a_O_state/1 -> E010A5_a_O_state_Term/1  "a_O_state"
  E010A5_fallback_state/1 -> E010A5_fallback_state_Term/1  "fallback_state"
  E010A5_burst_pulse_count_after_reentry/1 -> E010A5_burst_pulse_count_after_reentry_Term/1  "burst_pulse_count_after_reentry"
  E010A5_fallback_count/1 -> E010A5_fallback_count_Term/1  "fallback_count"
  E010A5_fallback_reason/1 -> E010A5_fallback_reason_Term/1  "fallback_reason"
  E010A5_TonActual_Clock/1 -> E010A5_TonActual1/2(t), E010A5_TonActual2/2(t), E010A5_TonActual3/2(t), E010A5_TonActual4/2(t)
  E010A5_TonActual1/1(Ton_actual) -> E010A5_TonActual1_Term/1  "Ton_actual1"
  E010A5_TonActual2/1(Ton_actual) -> E010A5_TonActual2_Term/1  "Ton_actual2"
  E010A5_TonActual3/1(Ton_actual) -> E010A5_TonActual3_Term/1  "Ton_actual3"
  E010A5_TonActual4/1(Ton_actual) -> E010A5_TonActual4_Term/1  "Ton_actual4"
  connections:
  DC Voltage Source/LConn1 -- Voltage Measurement1/LConn2 -- Mosfet7/RConn1 -- Voltage Measurement4/LConn2 -- DC Voltage Source3/LConn1 -- Mosfet6/RConn1 -- Voltage Measurement3/LConn2 -- DC Voltage Source2/LConn1 -- DC Voltage Source1/LConn1 -- Voltage Measurement2/LConn2 -- Mosfet5/RConn1 -- Voltage Measurement/LConn2 -- E010A5_Load_Current_Source/RConn1 -- Series RLC Branch4/RConn1 -- Mosfet4/RConn1 -- Ground/LConn1
  Mosfet/LConn1 -- DC Voltage Source/RConn1
  DC Voltage Source1/RConn1 -- Mosfet1/LConn1
  Mosfet1/RConn1 -- Current Measurement1/LConn1 -- Voltage Measurement2/LConn1
  DC Voltage Source2/RConn1 -- Mosfet2/LConn1
  Mosfet2/RConn1 -- Current Measurement2/LConn1 -- Voltage Measurement3/LConn1
  DC Voltage Source3/RConn1 -- Mosfet3/LConn1
  Series RLC Branch/RConn1 -- Series RLC Branch3/RConn1 -- Series RLC Branch2/RConn1 -- Series RLC Branch1/RConn1 -- Voltage Measurement/LConn1 -- E010A5_Load_Current_Source/LConn1 -- Series RLC Branch4/LConn1
  Mosfet/RConn1 -- Current Measurement/LConn1 -- Voltage Measurement1/LConn1
  Mosfet3/RConn1 -- Current Measurement3/LConn1 -- Voltage Measurement4/LConn1
  Current Measurement/RConn1 -- Mosfet4/LConn1 -- IL_Measurement1/LConn1
  IL_Measurement1/RConn1 -- Series RLC Branch/LConn1
  Current Measurement1/RConn1 -- Mosfet5/LConn1 -- IL_Measurement2/LConn1
  IL_Measurement2/RConn1 -- Series RLC Branch1/LConn1
  Mosfet6/LConn1 -- Current Measurement2/RConn1 -- IL_Measurement3/LConn1
  IL_Measurement3/RConn1 -- Series RLC Branch2/LConn1
  Current Measurement3/RConn1 -- Mosfet7/LConn1 -- IL_Measurement4/LConn1
  IL_Measurement4/RConn1 -- Series RLC Branch3/LConn1

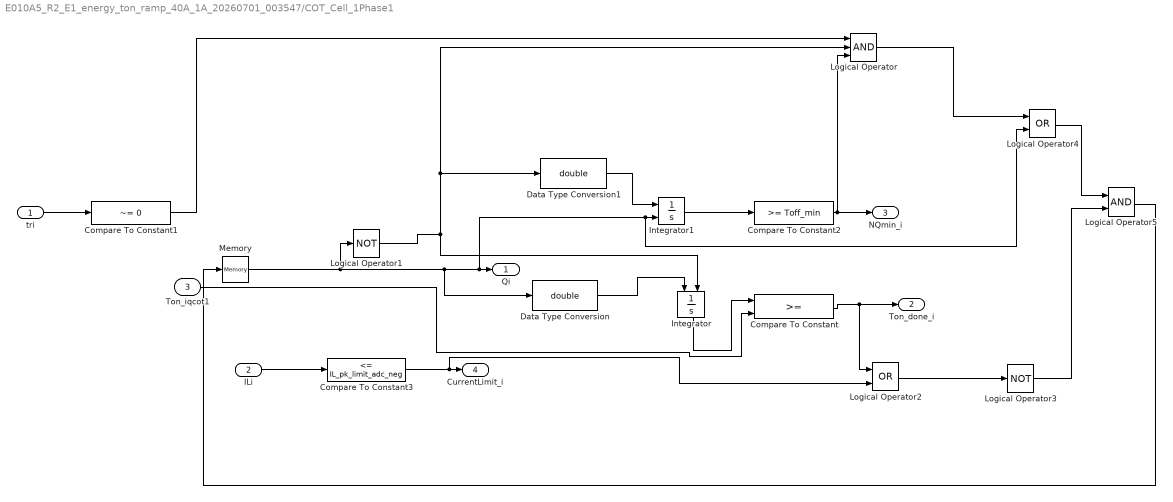
== system E010A5_R2_E1_energy_ton_ramp_40A_1A_20260701_003547/COT_Cell_1Phase1 ==
  tri : Inport
  ILi : Inport  Port=2
  Ton_iqcot1 : Inport  Port=3
  Compare To Constant : RelationalOperator  OutDataTypeStr=boolean  RndMeth=Simplest  InputSameDT=off
  Compare To Constant1 : simulink/Logic and Bit Operations/Compare To Constant  relop=~=  const=0  OutDataTypeStr=boolean
  Compare To Constant2 : simulink/Logic and Bit Operations/Compare To Constant  relop=>=  const=Toff_min  OutDataTypeStr=boolean
  Compare To Constant3 : simulink/Logic and Bit Operations/Compare To Constant  relop=<=  const=IL_pk_limit_adc_neg  OutDataTypeStr=boolean
  Data Type Conversion : DataTypeConversion  OutDataTypeStr=double  SaturateOnIntegerOverflow=off  RndMeth=Floor
  Data Type Conversion1 : DataTypeConversion  OutDataTypeStr=double  SaturateOnIntegerOverflow=off  RndMeth=Floor
  Integrator : Integrator  ExternalReset=level
  Integrator1 : Integrator  ExternalReset=level  InitialCondition=Toff_min
  Logical Operator : Logic  Inputs=3  AllPortsSameDT=off  OutDataTypeStr=boolean
  Logical Operator1 : Logic  Operator=NOT  AllPortsSameDT=off  OutDataTypeStr=boolean
  Logical Operator2 : Logic  Operator=OR  AllPortsSameDT=off  OutDataTypeStr=boolean
  Logical Operator3 : Logic  Operator=NOT  Inputs=3  AllPortsSameDT=off  OutDataTypeStr=boolean
  Logical Operator4 : Logic  Operator=OR  AllPortsSameDT=off  OutDataTypeStr=boolean
  Logical Operator5 : Logic  AllPortsSameDT=off  OutDataTypeStr=boolean
  Memory : Memory
  Qi : Outport
  Ton_done_i : Outport  Port=2
  NQmin_i : Outport  Port=3
  CurrentLimit_i : Outport  Port=4
  wires:
  Compare To Constant/1 -> Logical Operator2/1, Ton_done_i/1
  tri/1 -> Compare To Constant1/1
  Compare To Constant1/1 -> Logical Operator/1
  Memory/1 -> Logical Operator1/1, Data Type Conversion/1, Logical Operator4/2, Integrator1/2, Qi/1
  Logical Operator1/1 -> Data Type Conversion1/1, Logical Operator/2, Integrator/2
  Data Type Conversion/1 -> Integrator/1
  Integrator/1 -> Compare To Constant/1
  Data Type Conversion1/1 -> Integrator1/1
  Integrator1/1 -> Compare To Constant2/1
  Compare To Constant2/1 -> Logical Operator/3, NQmin_i/1
  ILi/1 -> Compare To Constant3/1
  Compare To Constant3/1 -> Logical Operator2/2, CurrentLimit_i/1
  Logical Operator2/1 -> Logical Operator3/1
  Logical Operator/1 -> Logical Operator4/1
  Logical Operator4/1 -> Logical Operator5/1
  Logical Operator3/1 -> Logical Operator5/2
  Logical Operator5/1 -> Memory/1
  Ton_iqcot1/1 -> Compare To Constant/2

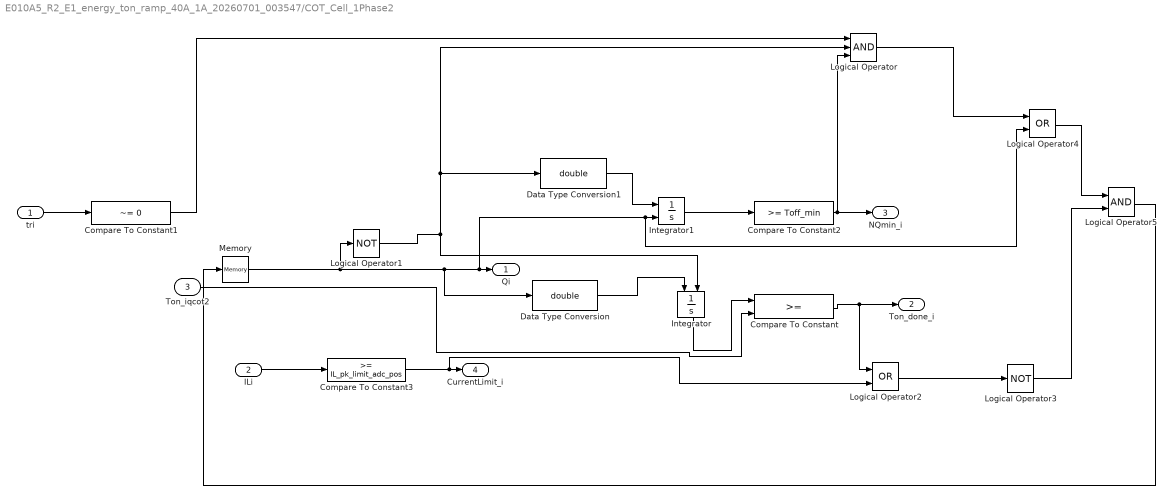
== system E010A5_R2_E1_energy_ton_ramp_40A_1A_20260701_003547/COT_Cell_1Phase2 ==
  tri : Inport
  ILi : Inport  Port=2
  Ton_iqcot2 : Inport  Port=3
  Compare To Constant : RelationalOperator  OutDataTypeStr=boolean  RndMeth=Simplest  InputSameDT=off
  Compare To Constant1 : simulink/Logic and Bit Operations/Compare To Constant  relop=~=  const=0  OutDataTypeStr=boolean
  Compare To Constant2 : simulink/Logic and Bit Operations/Compare To Constant  relop=>=  const=Toff_min  OutDataTypeStr=boolean
  Compare To Constant3 : simulink/Logic and Bit Operations/Compare To Constant  relop=>=  const=IL_pk_limit_adc_pos  OutDataTypeStr=boolean
  Data Type Conversion : DataTypeConversion  OutDataTypeStr=double  SaturateOnIntegerOverflow=off  RndMeth=Floor
  Data Type Conversion1 : DataTypeConversion  OutDataTypeStr=double  SaturateOnIntegerOverflow=off  RndMeth=Floor
  Integrator : Integrator  ExternalReset=level
  Integrator1 : Integrator  ExternalReset=level  InitialCondition=Toff_min
  Logical Operator : Logic  Inputs=3  AllPortsSameDT=off  OutDataTypeStr=boolean
  Logical Operator1 : Logic  Operator=NOT  AllPortsSameDT=off  OutDataTypeStr=boolean
  Logical Operator2 : Logic  Operator=OR  AllPortsSameDT=off  OutDataTypeStr=boolean
  Logical Operator3 : Logic  Operator=NOT  Inputs=3  AllPortsSameDT=off  OutDataTypeStr=boolean
  Logical Operator4 : Logic  Operator=OR  AllPortsSameDT=off  OutDataTypeStr=boolean
  Logical Operator5 : Logic  AllPortsSameDT=off  OutDataTypeStr=boolean
  Memory : Memory
  Qi : Outport
  Ton_done_i : Outport  Port=2
  NQmin_i : Outport  Port=3
  CurrentLimit_i : Outport  Port=4
  wires:
  Compare To Constant/1 -> Logical Operator2/1, Ton_done_i/1
  tri/1 -> Compare To Constant1/1
  Compare To Constant1/1 -> Logical Operator/1
  Memory/1 -> Logical Operator1/1, Data Type Conversion/1, Logical Operator4/2, Integrator1/2, Qi/1
  Logical Operator1/1 -> Data Type Conversion1/1, Logical Operator/2, Integrator/2
  Data Type Conversion/1 -> Integrator/1
  Integrator/1 -> Compare To Constant/1
  Data Type Conversion1/1 -> Integrator1/1
  Integrator1/1 -> Compare To Constant2/1
  Compare To Constant2/1 -> Logical Operator/3, NQmin_i/1
  ILi/1 -> Compare To Constant3/1
  Compare To Constant3/1 -> Logical Operator2/2, CurrentLimit_i/1
  Logical Operator2/1 -> Logical Operator3/1
  Logical Operator/1 -> Logical Operator4/1
  Logical Operator4/1 -> Logical Operator5/1
  Logical Operator3/1 -> Logical Operator5/2
  Logical Operator5/1 -> Memory/1
  Ton_iqcot2/1 -> Compare To Constant/2

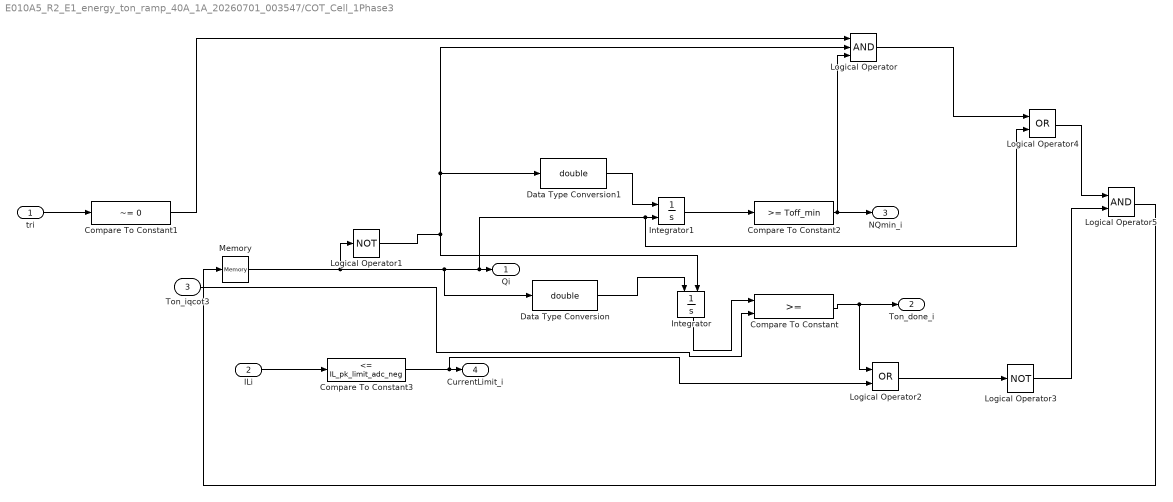
== system E010A5_R2_E1_energy_ton_ramp_40A_1A_20260701_003547/COT_Cell_1Phase3 ==
  tri : Inport
  ILi : Inport  Port=2
  Ton_iqcot3 : Inport  Port=3
  Compare To Constant : RelationalOperator  OutDataTypeStr=boolean  RndMeth=Simplest  InputSameDT=off
  Compare To Constant1 : simulink/Logic and Bit Operations/Compare To Constant  relop=~=  const=0  OutDataTypeStr=boolean
  Compare To Constant2 : simulink/Logic and Bit Operations/Compare To Constant  relop=>=  const=Toff_min  OutDataTypeStr=boolean
  Compare To Constant3 : simulink/Logic and Bit Operations/Compare To Constant  relop=<=  const=IL_pk_limit_adc_neg  OutDataTypeStr=boolean
  Data Type Conversion : DataTypeConversion  OutDataTypeStr=double  SaturateOnIntegerOverflow=off  RndMeth=Floor
  Data Type Conversion1 : DataTypeConversion  OutDataTypeStr=double  SaturateOnIntegerOverflow=off  RndMeth=Floor
  Integrator : Integrator  ExternalReset=level
  Integrator1 : Integrator  ExternalReset=level  InitialCondition=Toff_min
  Logical Operator : Logic  Inputs=3  AllPortsSameDT=off  OutDataTypeStr=boolean
  Logical Operator1 : Logic  Operator=NOT  AllPortsSameDT=off  OutDataTypeStr=boolean
  Logical Operator2 : Logic  Operator=OR  AllPortsSameDT=off  OutDataTypeStr=boolean
  Logical Operator3 : Logic  Operator=NOT  Inputs=3  AllPortsSameDT=off  OutDataTypeStr=boolean
  Logical Operator4 : Logic  Operator=OR  AllPortsSameDT=off  OutDataTypeStr=boolean
  Logical Operator5 : Logic  AllPortsSameDT=off  OutDataTypeStr=boolean
  Memory : Memory
  Qi : Outport
  Ton_done_i : Outport  Port=2
  NQmin_i : Outport  Port=3
  CurrentLimit_i : Outport  Port=4
  wires:
  Compare To Constant/1 -> Logical Operator2/1, Ton_done_i/1
  tri/1 -> Compare To Constant1/1
  Compare To Constant1/1 -> Logical Operator/1
  Memory/1 -> Logical Operator1/1, Data Type Conversion/1, Logical Operator4/2, Integrator1/2, Qi/1
  Logical Operator1/1 -> Data Type Conversion1/1, Logical Operator/2, Integrator/2
  Data Type Conversion/1 -> Integrator/1
  Integrator/1 -> Compare To Constant/1
  Data Type Conversion1/1 -> Integrator1/1
  Integrator1/1 -> Compare To Constant2/1
  Compare To Constant2/1 -> Logical Operator/3, NQmin_i/1
  ILi/1 -> Compare To Constant3/1
  Compare To Constant3/1 -> Logical Operator2/2, CurrentLimit_i/1
  Logical Operator2/1 -> Logical Operator3/1
  Logical Operator/1 -> Logical Operator4/1
  Logical Operator4/1 -> Logical Operator5/1
  Logical Operator3/1 -> Logical Operator5/2
  Logical Operator5/1 -> Memory/1
  Ton_iqcot3/1 -> Compare To Constant/2

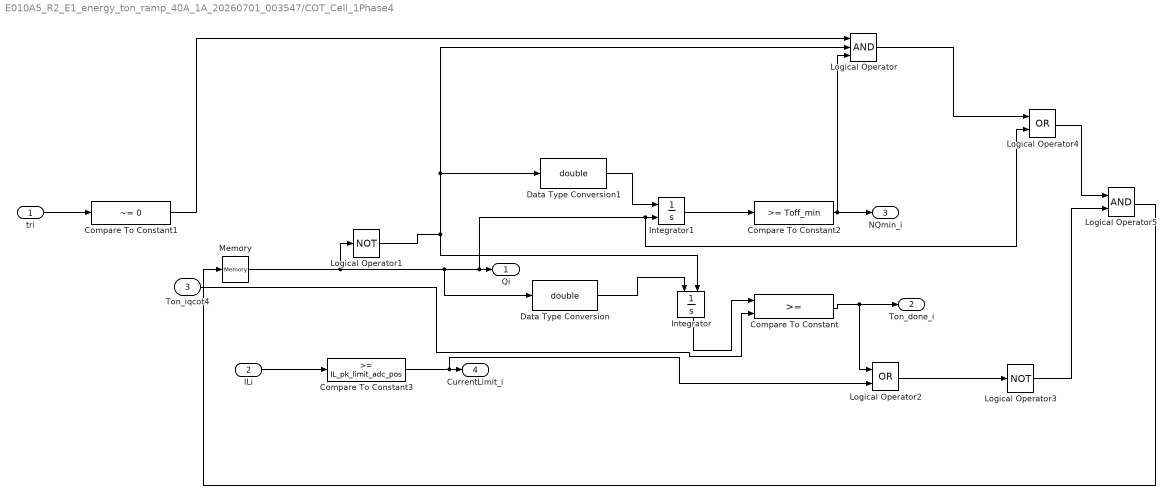
== system E010A5_R2_E1_energy_ton_ramp_40A_1A_20260701_003547/COT_Cell_1Phase4 ==
  tri : Inport
  ILi : Inport  Port=2
  Ton_iqcot4 : Inport  Port=3
  Compare To Constant : RelationalOperator  OutDataTypeStr=boolean  RndMeth=Simplest  InputSameDT=off
  Compare To Constant1 : simulink/Logic and Bit Operations/Compare To Constant  relop=~=  const=0  OutDataTypeStr=boolean
  Compare To Constant2 : simulink/Logic and Bit Operations/Compare To Constant  relop=>=  const=Toff_min  OutDataTypeStr=boolean
  Compare To Constant3 : simulink/Logic and Bit Operations/Compare To Constant  relop=>=  const=IL_pk_limit_adc_pos  OutDataTypeStr=boolean
  Data Type Conversion : DataTypeConversion  OutDataTypeStr=double  SaturateOnIntegerOverflow=off  RndMeth=Floor
  Data Type Conversion1 : DataTypeConversion  OutDataTypeStr=double  SaturateOnIntegerOverflow=off  RndMeth=Floor
  Integrator : Integrator  ExternalReset=level
  Integrator1 : Integrator  ExternalReset=level  InitialCondition=Toff_min
  Logical Operator : Logic  Inputs=3  AllPortsSameDT=off  OutDataTypeStr=boolean
  Logical Operator1 : Logic  Operator=NOT  AllPortsSameDT=off  OutDataTypeStr=boolean
  Logical Operator2 : Logic  Operator=OR  AllPortsSameDT=off  OutDataTypeStr=boolean
  Logical Operator3 : Logic  Operator=NOT  Inputs=3  AllPortsSameDT=off  OutDataTypeStr=boolean
  Logical Operator4 : Logic  Operator=OR  AllPortsSameDT=off  OutDataTypeStr=boolean
  Logical Operator5 : Logic  AllPortsSameDT=off  OutDataTypeStr=boolean
  Memory : Memory
  Qi : Outport
  Ton_done_i : Outport  Port=2
  NQmin_i : Outport  Port=3
  CurrentLimit_i : Outport  Port=4
  wires:
  Compare To Constant/1 -> Logical Operator2/1, Ton_done_i/1
  tri/1 -> Compare To Constant1/1
  Compare To Constant1/1 -> Logical Operator/1
  Memory/1 -> Logical Operator1/1, Data Type Conversion/1, Logical Operator4/2, Integrator1/2, Qi/1
  Logical Operator1/1 -> Data Type Conversion1/1, Logical Operator/2, Integrator/2
  Data Type Conversion/1 -> Integrator/1
  Integrator/1 -> Compare To Constant/1
  Data Type Conversion1/1 -> Integrator1/1
  Integrator1/1 -> Compare To Constant2/1
  Compare To Constant2/1 -> Logical Operator/3, NQmin_i/1
  ILi/1 -> Compare To Constant3/1
  Compare To Constant3/1 -> Logical Operator2/2, CurrentLimit_i/1
  Logical Operator2/1 -> Logical Operator3/1
  Logical Operator/1 -> Logical Operator4/1
  Logical Operator4/1 -> Logical Operator5/1
  Logical Operator3/1 -> Logical Operator5/2
  Logical Operator5/1 -> Memory/1
  Ton_iqcot4/1 -> Compare To Constant/2

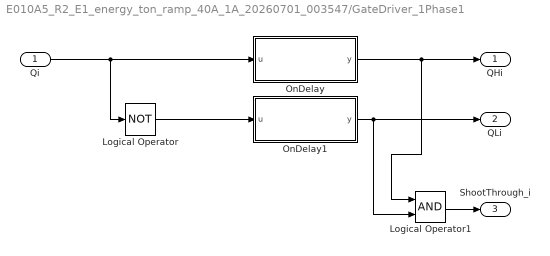
== system E010A5_R2_E1_energy_ton_ramp_40A_1A_20260701_003547/GateDriver_1Phase1 ==
  Qi : Inport
  Logical Operator : Logic  Operator=NOT  AllPortsSameDT=off  OutDataTypeStr=boolean
  Logical Operator1 : Logic  AllPortsSameDT=off  OutDataTypeStr=boolean
  OnDelay : Subsystem
  OnDelay1 : Subsystem
  QHi : Outport
  QLi : Outport  Port=2
  ShootThrough_i : Outport  Port=3
  wires:
  Qi/1 -> Logical Operator/1, OnDelay/1(u)
  OnDelay/1(y) -> Logical Operator1/1, QHi/1
  Logical Operator/1 -> OnDelay1/1(u)
  OnDelay1/1(y) -> QLi/1, Logical Operator1/2
  Logical Operator1/1 -> ShootThrough_i/1

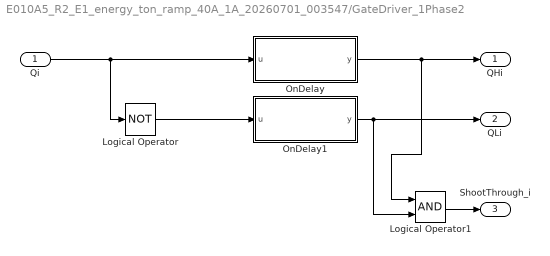
== system E010A5_R2_E1_energy_ton_ramp_40A_1A_20260701_003547/GateDriver_1Phase2 ==
  Qi : Inport
  Logical Operator : Logic  Operator=NOT  AllPortsSameDT=off  OutDataTypeStr=boolean
  Logical Operator1 : Logic  AllPortsSameDT=off  OutDataTypeStr=boolean
  OnDelay : Subsystem
  OnDelay1 : Subsystem
  QHi : Outport
  QLi : Outport  Port=2
  ShootThrough_i : Outport  Port=3
  wires:
  Qi/1 -> Logical Operator/1, OnDelay/1(u)
  OnDelay/1(y) -> Logical Operator1/1, QHi/1
  Logical Operator/1 -> OnDelay1/1(u)
  OnDelay1/1(y) -> QLi/1, Logical Operator1/2
  Logical Operator1/1 -> ShootThrough_i/1

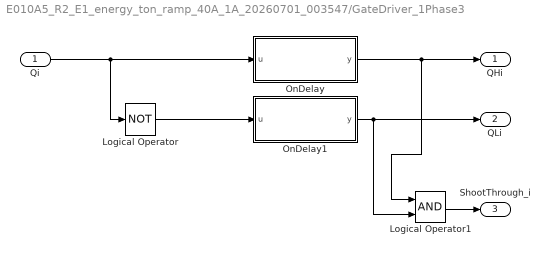
== system E010A5_R2_E1_energy_ton_ramp_40A_1A_20260701_003547/GateDriver_1Phase3 ==
  Qi : Inport
  Logical Operator : Logic  Operator=NOT  AllPortsSameDT=off  OutDataTypeStr=boolean
  Logical Operator1 : Logic  AllPortsSameDT=off  OutDataTypeStr=boolean
  OnDelay : Subsystem
  OnDelay1 : Subsystem
  QHi : Outport
  QLi : Outport  Port=2
  ShootThrough_i : Outport  Port=3
  wires:
  Qi/1 -> Logical Operator/1, OnDelay/1(u)
  OnDelay/1(y) -> Logical Operator1/1, QHi/1
  Logical Operator/1 -> OnDelay1/1(u)
  OnDelay1/1(y) -> QLi/1, Logical Operator1/2
  Logical Operator1/1 -> ShootThrough_i/1
